simulink model "BANSHEE_20161130"  (Simulink 8.1)
settings: Solver=ode1  StartTime=0.0  StopTime=inf  FixedStep=Ts  MaxStep=1e-3  RelTol=1e-3
PostLoadFcn:
  | BANSHEE_init;
InitFcn:
  | BANSHEE_init;
values from neighbouring files (symbols this model uses):
  F1 = xlsread('F1_relay_banshee.xlsx')    [relay_settings_init.m]
  F2 = xlsread('F2_relay_banshee.xlsx')    [relay_settings_init.m]
  F3 = xlsread('F3_relay_banshee.xlsx')    [relay_settings_init.m]
  Ts = 100E-6    (= 0.0001)    [BANSHEE_init.m]
undefined symbols (not defined in the file or in its folder): cable_spec, fdesignblkfcn, Feeder1_lib, Feeder2_lib, Feeder3_lib, gcbh, generic_ethernet_cb, Left, relay_housing_lib, SM_UtilityService, SS_F1_RELAY_HOUSING, SS_F2_RELAY_HOUSING, SS_F3_RELAY_HOUSING, SS_Feeder1, SS_Feeder2, SS_Feeder3, type, utility_service_lib, V
libraries: breaker_lib x47, rtio_generic_modbus x43, relay_modbus_lib x42, cables_lib x38, transformer_lib x22, Load_lib x20, artemis x18, powerlib x18, rtio_opalrt_common x15, ssn_lib x15, rtlab x14, simulink x10
(part 3 of 5)

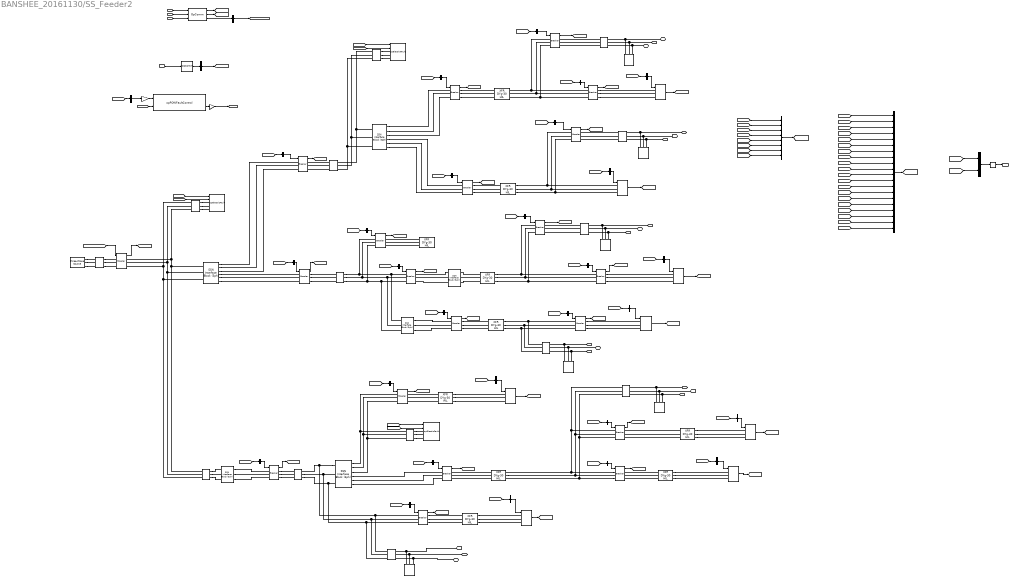
== system BANSHEE_20161130/SS_Feeder2 ==
  note: connect to F1
  note: connect to F1
  note: connect to F3
  note: connect to F3
  note: connect to F3
  note: BATT SYSTEM
  note: PV SYSTEM
  note: connect to F1
  note: % Copyright (c) 2016 Massachusetts Institute of Technology
      | % Permission is hereby granted, free of charge, to any person obtaining a copy of this
      | % software and associated documentation files (the "Software"), to deal in the Software
      | % without restriction, including without limitation the rights to use, copy, modify,
      | % merge, publish, distribute, sublicense, and/or sell copies of the Software, and to
      | % permit persons to whom the Software is furnished to do so, subject to the following
      | % conditions:
      | %
      | %
      | % The above copyright notice and this permission notice shall be included in
      | % all copies or substantial portions of the Software.
      | %
      | % THE SOFTWARE IS PROVIDED "AS IS", WITHOUT WARRANTY OF ANY KIND, EXPRESS OR IMPLIED,
      | % INCLUDING BUT NOT LIMITED TO THE WARRANTIES OF MERCHANTABILITY, FITNESS FOR A
      | % PARTICULAR PURPOSE AND NONINFRINGEMENT. IN NO EVENT SHALL THE AUTHORS OR COPYRIGHT
      | % HOLDERS BE LIABLE FOR ANY CLAIM, DAMAGES OR OTHER LIABILITY, WHETHER IN AN ACTION
      | % OF CONTRACT, TORT OR OTHERWISE, ARISING FROM, OUT OF OR IN CONNECTION WITH THE
      | % SOFTWARE OR THE USE OR OTHER DEALINGS IN THE SOFTWARE.
      | %
      | %
      | %%
  note: Point-on-wave synchronisation voltage (3-phase) in PU - Using 13.8 kV
  RELAY_IN : Inport
  LOAD_IN : Inport  Port=2
  SC_CMD : Inport  Port=3
  HWCtrl_CMD : Inport  Port=4
  1000 kVA1 : transformer_lib/XFR DYg-30 HIL  Rating=1000  Vp=13800  Vs=480  Z=5.56  XR=4.49
  1000 kVA2 : transformer_lib/XFR DYg-30 HIL  Rating=1000  Vp=13800  Vs=480  Z=5.56  XR=5.49
  1270 kvar inductor at 13.8kV  to cancel kvar produced by the stublines1 : powerlib/Elements/Three-Phase Parallel RLC Load  LConnTagsString=A|B|C  Configuration=Y (grounded)  NominalVoltage=13800  NominalFrequency=60  ActivePower=0  InductivePower=1270e3  CapacitivePower=0  Measurements=None  LoadType=constant Z
  1500 kVA : transformer_lib/XFR DYg-30 HIL  Rating=1500  Vp=13800  Vs=480  Z=5.56  XR=5.51
  2000 kVA2 : transformer_lib/XFR DYg-30 HIL  Rating=2000  Vp=13800  Vs=480  Z=5.75  XR=5.7
  2000 kVA3 : transformer_lib/XFR DYg-30 HIL  Rating=2000  Vp=13800  Vs=480  Z=5.75  XR=5.7
  2500 kVA : transformer_lib/XFR DYg-30 HIL  Rating=2500  Vp=13800  Vs=480  Z=5.56  XR=5.52
  2500 kVA1 : transformer_lib/XFR DYg-30 HIL  Rating=2500  Vp=13800  Vs=480  Z=5.56  XR=5.52
  346 kvar inductor at 4160V  to cancel kvar produced by the stublines5 : powerlib/Elements/Three-Phase Parallel RLC Load  LConnTagsString=A|B|C  Configuration=Y (grounded)  NominalVoltage=4160  NominalFrequency=60  ActivePower=0  InductivePower=346e3  CapacitivePower=0  Measurements=None  LoadType=constant Z
  3750 kVA : transformer_lib/XFR DYg-30 HIL  Rating=3750  Vp=13800  Vs=4160  Z=4.75  XR=11.4
  500 kVA : transformer_lib/XFR DYg-30 HIL  Rating=500  Vp=13800  Vs=208  Z=5  XR=4.9
  5000 kVA : transformer_lib/XFR DYg-30 HIL  Rating=5000  Vp=13800  Vs=480  Z=5.50  XR=5.44
  500kcmil_cable : cables_lib/500kcmil_cable  length=1  par_sets=1
  500kcmil_cable1 : cables_lib/500kcmil_cable  length=1  par_sets=1
  500kcmil_cable2 : cables_lib/500kcmil_cable  length=1  par_sets=1
  6 kvar inductor at 480V  to cancel kvar produced by the stublines1 : powerlib/Elements/Three-Phase Parallel RLC Load  LConnTagsString=A|B|C  Configuration=Y (grounded)  NominalVoltage=480  NominalFrequency=60  ActivePower=0  InductivePower=6e3  CapacitivePower=0  Measurements=None  LoadType=constant Z
  6 kvar inductor at 480V  to cancel kvar produced by the stublines2 : powerlib/Elements/Three-Phase Parallel RLC Load  LConnTagsString=A|B|C  Configuration=Y (grounded)  NominalVoltage=480  NominalFrequency=60  ActivePower=0  InductivePower=6e3  CapacitivePower=0  Measurements=None  LoadType=constant Z
  6 kvar inductor at 480V  to cancel kvar produced by the stublines3 : powerlib/Elements/Three-Phase Parallel RLC Load  LConnTagsString=A|B|C  Configuration=Y (grounded)  NominalVoltage=480  NominalFrequency=60  ActivePower=0  InductivePower=6e3  CapacitivePower=0  Measurements=None  LoadType=constant Z
  6 kvar inductor at 480V  to cancel kvar produced by the stublines4 : powerlib/Elements/Three-Phase Parallel RLC Load  LConnTagsString=A|B|C  Configuration=Y (grounded)  NominalVoltage=480  NominalFrequency=60  ActivePower=0  InductivePower=9e3  CapacitivePower=0  Measurements=None  LoadType=constant Z
  Bus Creator2 : BusCreator  Inputs=2
  Bus Creator3 : BusCreator  Inputs=8
  Bus Creator5 : BusCreator  Inputs=20
  Bus Selector : BusSelector  OutputSignals=Vabc_bus
  Bus Selector1 : BusSelector  OutputSignals=F2_CB_4
  Bus Selector10 : BusSelector  OutputSignals=I4
  Bus Selector11 : BusSelector  OutputSignals=F2_CB_11
  Bus Selector12 : BusSelector  OutputSignals=F2_CB_15
  Bus Selector13 : BusSelector  OutputSignals=F2_CB_3
  Bus Selector14 : BusSelector  OutputSignals=F2_CB_14
  Bus Selector15 : BusSelector  OutputSignals=F2_CB_17
  Bus Selector16 : BusSelector  OutputSignals=F2_CB_16
  Bus Selector17 : BusSelector  OutputSignals=F2_CB_13
  Bus Selector18 : BusSelector  OutputSignals=F2_CB_10
  Bus Selector19 : BusSelector  OutputSignals=F2_CB_9
  Bus Selector2 : BusSelector  OutputSignals=F2_CB_2
  Bus Selector20 : BusSelector  OutputSignals=F2_CB_12
  Bus Selector21 : BusSelector  OutputSignals=F2_CB_5
  Bus Selector22 : BusSelector  OutputSignals=F2_CB_7
  Bus Selector23 : BusSelector  OutputSignals=F2_CB_8
  Bus Selector24 : BusSelector  OutputSignals=F2_CB_6
  Bus Selector25 : BusSelector  OutputSignals=F2_CB_1
  Bus Selector26 : BusSelector  OutputSignals=F2_CB_18
  Bus Selector27 : BusSelector  OutputSignals=F2_CB_19
  Bus Selector28 : BusSelector  OutputSignals=fault_cmd
  Bus Selector29 : BusSelector  OutputSignals=SEL751_LogicTrip.F2.Logic_trip
  Bus Selector3 : BusSelector  OutputSignals=P5
  Bus Selector4 : BusSelector  OutputSignals=C4
  Bus Selector5 : BusSelector  OutputSignals=I5
  Bus Selector6 : BusSelector  OutputSignals=P2
  Bus Selector7 : BusSelector  OutputSignals=C3
  Bus Selector8 : BusSelector  OutputSignals=P3
  Bus Selector9 : BusSelector  OutputSignals=I3
  C1 : cables_lib/PI-Section  cable_spec=[cable_spec(11, :)]  line_length=10  parallel_sets=1
  C{2..4,204..206} (6 alike) : cables_lib/PI-Section  cable_spec=[cable_spec(6, :)]  line_length=10  parallel_sets=1
  C201 : cables_lib/PI-Section  cable_spec=[cable_spec(11, :)]  line_length=5500  parallel_sets=1
  C202 : cables_lib/PI-Section  cable_spec=[cable_spec(13, :)]  line_length=2000  parallel_sets=1
  C203 : cables_lib/PI-Section  cable_spec=[cable_spec(13, :)]  line_length=3000  parallel_sets=1
  Critical_3 : Load_lib/Dynamic_Load  V=460  Ts=Ts
  Critical_4 : Load_lib/Dynamic_Load  V=460  Ts=Ts
  F2_CB_{1..19} (19 alike) : breaker_lib/Breaker  Ts=Ts  mech_delay=cb_mech_delay
  F2_PCC : breaker_lib/Breaker  Ts=Ts  mech_delay=cb_mech_delay
  Interruptible_3 : Load_lib/Dynamic_Load  V=208  Ts=Ts
  Interruptible_4 : Load_lib/Dynamic_Load  V=460  Ts=Ts
  Interruptible_5 : Load_lib/Dynamic_Load  V=460  Ts=Ts
  Memory : Memory
  OpComm1 : rtlab/OpComm  nbport=3  groupe_acq=1  subsys_rate=0  st=0  Synchronization=on  Interpolation=on  Threshold=1.0  Missed_Data=off  Sim_Time=off  Samples=off  dynSigOut=off  from_console=0  warning_done=off  writeOpCommFile=off  Offset=off
  OpComm2 : rtlab/OpComm  nbport=1  groupe_acq=1  subsys_rate=0  st=0  Synchronization=on  Interpolation=on  Threshold=1.0  Missed_Data=off  Sim_Time=off  Samples=off  dynSigOut=off  from_console=1  warning_done=off  writeOpCommFile=off  Offset=off
  PI-Section1 : cables_lib/PI-Section  cable_spec=[cable_spec(13, :)]  line_length=500  parallel_sets=1
  Priority_2 : Load_lib/Dynamic_Load  V=460  Ts=Ts
  Priority_3 : Load_lib/Dynamic_Load  V=460  Ts=Ts
  Priority_5 : Load_lib/Dynamic_Load  V=460  Ts=Ts
  SSN Interface Block (3ph)1 : ssn_lib/SSN Interface Block (3ph)  nb_phase=3  nb_port=3  p1_type=V-type(Left)  p2_type=V-type (Right)  p3_type=V-type (Right)  p4_type=V-type(Left)  p5_type=V-type(Left)  p6_type=V-type(Left)  p7_type=V-type(Left)  p8_type=V-type(Left)  p9_type=V-type(Left)  p10_type=V-type(Left)  p11_type=V-type(Left)  p12_type=V-type(Left)  p13_type=V-type(Left)  p14_type=V-type(Left)  p15_type=V-type(Left)  p16_type=V-type(Left)  I_port_shunt_resistance=1e9
  SSN Interface Block (3ph)10 : ssn_lib/SSN Interface Block (3ph)  nb_phase=3  nb_port=2  p1_type=V-type(Left)  p2_type=V-type (Right)  p3_type=V-type(Left)  p4_type=V-type(Left)  p5_type=V-type(Left)  p6_type=V-type(Left)  p7_type=V-type(Left)  p8_type=V-type(Left)  p9_type=V-type(Left)  p10_type=V-type(Left)  p11_type=V-type(Left)  p12_type=V-type(Left)  p13_type=V-type(Left)  p14_type=V-type(Left)  p15_type=V-type(Left)  p16_type=V-type(Left)  I_port_shunt_resistance=1e9
  SSN Interface Block (3ph)2 : ssn_lib/SSN Interface Block (3ph)  nb_phase=3  nb_port=3  p1_type=V-type(Left)  p2_type=V-type (Right)  p3_type=V-type (Right)  p4_type=V-type(Left)  p5_type=V-type(Left)  p6_type=V-type(Left)  p7_type=V-type(Left)  p8_type=V-type(Left)  p9_type=V-type(Left)  p10_type=V-type(Left)  p11_type=V-type(Left)  p12_type=V-type(Left)  p13_type=V-type(Left)  p14_type=V-type(Left)  p15_type=V-type(Left)  p16_type=V-type(Left)  I_port_shunt_resistance=1e9
  SSN Interface Block (3ph)3 : ssn_lib/SSN Interface Block (3ph)  nb_phase=3  nb_port=2  p1_type=V-type(Left)  p2_type=V-type (Right)  p3_type=V-type(Left)  p4_type=V-type(Left)  p5_type=V-type(Left)  p6_type=V-type(Left)  p7_type=V-type(Left)  p8_type=V-type(Left)  p9_type=V-type(Left)  p10_type=V-type(Left)  p11_type=V-type(Left)  p12_type=V-type(Left)  p13_type=V-type(Left)  p14_type=V-type(Left)  p15_type=V-type(Left)  p16_type=V-type(Left)  I_port_shunt_resistance=1e9
  SSN Interface Block (3ph)4 : ssn_lib/SSN Interface Block (3ph)  nb_phase=3  nb_port=3  p1_type=V-type(Left)  p2_type=V-type (Right)  p3_type=V-type (Right)  p4_type=V-type(Left)  p5_type=V-type(Left)  p6_type=V-type(Left)  p7_type=V-type(Left)  p8_type=V-type(Left)  p9_type=V-type(Left)  p10_type=V-type(Left)  p11_type=V-type(Left)  p12_type=V-type(Left)  p13_type=V-type(Left)  p14_type=V-type(Left)  p15_type=V-type(Left)  p16_type=V-type(Left)  I_port_shunt_resistance=1e9
  SSN Interface Block (3ph)9 : ssn_lib/SSN Interface Block (3ph)  nb_phase=3  nb_port=2  p1_type=V-type(Left)  p2_type=V-type (Right)  p3_type=V-type(Left)  p4_type=V-type(Left)  p5_type=V-type(Left)  p6_type=V-type(Left)  p7_type=V-type(Left)  p8_type=V-type(Left)  p9_type=V-type(Left)  p10_type=V-type(Left)  p11_type=V-type(Left)  p12_type=V-type(Left)  p13_type=V-type(Left)  p14_type=V-type(Left)  p15_type=V-type(Left)  p16_type=V-type(Left)  I_port_shunt_resistance=1e9
  Three-Phase Source1 : powerlib/Electrical Sources/Three-Phase Source  Voltage=13800  PhaseAngle=0  Frequency=60  InternalConnection=Yg  SpecifyImpedance=on  Resistance=0.8929  Inductance=16.58e-3  ShortCircuitLevel=375e6  BaseVoltage=13800  XRratio=5.2  BusType=swing  Pref=0  Qref=0  Qmin=-inf  Qmax=inf
  a : Gain  Gain=1/(13800*sqrt(2/3))
  opElectricFault : artemis/Tools /POW faults/opElectricFault  FaultLocation=location 5  FaultResistance=0.0001  GroundResistance=0.0001  InitialStates=[0 0 0]  SnubberResistance=1e6  SnubberCapacitance=inf
  opElectricFault1 : artemis/Tools /POW faults/opElectricFault  FaultLocation=location 1  FaultResistance=0.0001  GroundResistance=0.0001  InitialStates=[0 0 0]  SnubberResistance=1e6  SnubberCapacitance=inf
  opElectricFault2 : artemis/Tools /POW faults/opElectricFault  FaultLocation=location 6  FaultResistance=0.0001  GroundResistance=0.0001  InitialStates=[0 0 0]  SnubberResistance=1e6  SnubberCapacitance=inf
  opPOWFaultControl1 : artemis/Tools /POW faults/opPOWFaultControl  Ts=Ts  usePLL=off  Fgrid=60  PLL_k=[180 3200 1]  vol_sel=1: rising zero-corssing  SyncPhase_menu=A  T_acq=0.8
  triggerFAULT : Gain
  A_CB_13 : PMIOPort  Port=1  Side=Right
  B_CB_13 : PMIOPort  Port=2  Side=Right
  C_CB_13 : PMIOPort  Port=3  Side=Right
  A_CB_17 : PMIOPort  Port=4  Side=Right
  B_CB_17 : PMIOPort  Port=5  Side=Right
  C_CB_17 : PMIOPort  Port=6  Side=Right
  A_CB_16 : PMIOPort  Port=7  Side=Right
  B_CB_16 : PMIOPort  Port=8  Side=Right
  C_CB_16 : PMIOPort  Port=9  Side=Right
  A_CB_9 : PMIOPort  Port=10  Side=Right
  B_CB_9 : PMIOPort  Port=11  Side=Right
  C_CB_9 : PMIOPort  Port=12  Side=Right
  A_CB_7 : PMIOPort  Port=13  Side=Right
  B_CB_7 : PMIOPort  Port=14  Side=Right
  C_CB_7 : PMIOPort  Port=15  Side=Right
  A_CB_1 : PMIOPort  Port=16  Side=Right
  B_CB_1 : PMIOPort  Port=17  Side=Right
  C_CB_1 : PMIOPort  Port=18  Side=Right
  DATA_OUT : Outport
  wires:
  LOAD_IN/1 -> OpComm1/1
  OpComm1/1 -> [LOAD_IN]
  [LOAD_IN] -> Bus Selector3/1
  [LOAD_IN] -> Bus Selector4/1
  [LOAD_IN] -> Bus Selector5/1
  [LOAD_IN] -> Bus Selector6/1
  [LOAD_IN] -> Bus Selector7/1
  [LOAD_IN] -> Bus Selector8/1
  [LOAD_IN] -> Bus Selector9/1
  [LOAD_IN] -> Bus Selector10/1
  Bus Selector3/1 -> Priority_5/1  "<P5>"
  Bus Selector4/1 -> Critical_4/1  "<C4>"
  Bus Selector5/1 -> Interruptible_5/1  "<I5>"
  Bus Selector6/1 -> Priority_2/1  "<P2>"
  Bus Selector7/1 -> Critical_3/1  "<C3>"
  Bus Selector8/1 -> Priority_3/1  "<P3>"
  Bus Selector10/1 -> Interruptible_4/1  "<I4>"
  Bus Selector9/1 -> Interruptible_3/1  "<I3>"
  Critical_4/1 -> [LOAD_C4]
  Priority_5/1 -> [LOAD_P5]
  Interruptible_5/1 -> [LOAD_I5]
  Priority_2/1 -> [LOAD_P2]
  Critical_3/1 -> [LOAD_C3]
  Interruptible_3/1 -> [LOAD_I3]
  Priority_3/1 -> [LOAD_P3]
  Interruptible_4/1 -> [LOAD_I4]
  [LOAD_C3] -> Bus Creator3/1  "F2_C3"
  Bus Creator3/1 -> [LOAD_DATA]  "LOAD"
  [LOAD_I4] -> Bus Creator3/4  "F2_I4"
  [LOAD_P2] -> Bus Creator3/6  "F2_P2"
  [LOAD_I5] -> Bus Creator3/5  "F2_I5"
  [LOAD_C4] -> Bus Creator3/2  "F2_C4"
  [LOAD_I3] -> Bus Creator3/3  "F2_I3"
  [LOAD_P3] -> Bus Creator3/7  "F2_P3"
  [LOAD_P5] -> Bus Creator3/8  "F2_P5"
  F2_CB_2/1 -> [F2_CB_2]
  F2_CB_1/1 -> [F2_CB_1]
  F2_CB_6/1 -> [F2_CB_6]
  F2_CB_7/1 -> [F2_CB_7]
  F2_CB_5/1 -> [F2_CB_5]
  F2_CB_8/1 -> [F2_CB_8]
  F2_CB_9/1 -> [F2_CB_9]
  F2_CB_3/1 -> [F2_CB_3]
  F2_CB_11/1 -> [F2_CB_11]
  F2_CB_15/1 -> [F2_CB_15]
  F2_CB_17/1 -> [F2_CB_17]
  F2_CB_14/1 -> [F2_CB_14]
  F2_CB_10/1 -> [F2_CB_10]
  F2_CB_13/1 -> [F2_CB_13]
  [F2_CB_1] -> Bus Creator5/1  "F2_CB_1"
  [F2_CB_2] -> Bus Creator5/2  "F2_CB_2"
  [F2_CB_3] -> Bus Creator5/3  "F2_CB_3"
  [F2_CB_6] -> Bus Creator5/6  "F2_CB_6"
  [F2_CB_4] -> Bus Creator5/4  "F2_CB_4"
  [F2_CB_9] -> Bus Creator5/9  "F2_CB_9"
  [F2_CB_7] -> Bus Creator5/7  "F2_CB_7"
  [F2_CB_11] -> Bus Creator5/11  "F2_CB_11"
  [F2_CB_14] -> Bus Creator5/14  "F2_CB_14"
  [F2_CB_5] -> Bus Creator5/5  "F2_CB_5"
  [F2_CB_8] -> Bus Creator5/8  "F2_CB_8"
  [F2_CB_12] -> Bus Creator5/12  "F2_CB_12"
  [F2_CB_10] -> Bus Creator5/10  "F2_CB_10"
  [F2_CB_13] -> Bus Creator5/13  "F2_CB_13"
  [F2_CB_15] -> Bus Creator5/15  "F2_CB_15"
  [F2_CB_16] -> Bus Creator5/16  "F2_CB_16"
  RELAY_IN/1 -> OpComm1/2
  OpComm1/2 -> [RELAY_IN]
  Bus Selector13/1 -> F2_CB_3/1  "<F2_CB_3>"
  [RELAY_IN] -> Bus Selector13/1
  [RELAY_IN] -> Bus Selector2/1
  [RELAY_IN] -> Bus Selector11/1
  [RELAY_IN] -> Bus Selector12/1
  [RELAY_IN] -> Bus Selector14/1
  [RELAY_IN] -> Bus Selector15/1
  [RELAY_IN] -> Bus Selector16/1
  [RELAY_IN] -> Bus Selector17/1
  [RELAY_IN] -> Bus Selector18/1
  [RELAY_IN] -> Bus Selector19/1
  [RELAY_IN] -> Bus Selector20/1
  [RELAY_IN] -> Bus Selector21/1
  [RELAY_IN] -> Bus Selector22/1
  [RELAY_IN] -> Bus Selector23/1
  [RELAY_IN] -> Bus Selector24/1
  [RELAY_IN] -> Bus Selector25/1
  Bus Selector2/1 -> F2_CB_2/1  "<F2_CB_2>"
  Bus Selector11/1 -> F2_CB_11/1  "<F2_CB_11>"
  Bus Selector18/1 -> F2_CB_10/1  "<F2_CB_10>"
  Bus Selector19/1 -> F2_CB_9/1  "<F2_CB_9>"
  Bus Selector17/1 -> F2_CB_13/1  "<F2_CB_13>"
  Bus Selector20/1 -> F2_CB_12/1  "<F2_CB_12>"
  Bus Selector14/1 -> F2_CB_14/1  "<F2_CB_14>"
  Bus Selector16/1 -> F2_CB_16/1  "<F2_CB_16>"
  Bus Selector12/1 -> F2_CB_15/1  "<F2_CB_15>"
  Bus Selector25/1 -> F2_CB_1/1  "<F2_CB_1>"
  Bus Selector21/1 -> F2_CB_5/1  "<F2_CB_5>"
  Bus Selector22/1 -> F2_CB_7/1  "<F2_CB_7>"
  Bus Selector24/1 -> F2_CB_6/1  "<F2_CB_6>"
  Bus Selector23/1 -> F2_CB_8/1  "<F2_CB_8>"
  [F2_CB_17] -> Bus Creator5/17  "F2_CB_17"
  Bus Selector15/1 -> F2_CB_17/1  "<F2_CB_17>"
  F2_CB_12/1 -> [F2_CB_12]
  F2_CB_16/1 -> [F2_CB_16]
  F2_PCC/1 -> [F2_PCC]
  [F2_PCC] -> Bus Creator5/20  "F2_PCC"
  F2_CB_4/1 -> [F2_CB_4]
  [RELAY_IN] -> Bus Selector1/1
  Bus Selector1/1 -> F2_CB_4/1  "<F2_CB_4>"
  F2_CB_18/1 -> [F2_CB_18]
  [RELAY_IN] -> Bus Selector26/1
  Bus Selector26/1 -> F2_CB_18/1  "<F2_CB_18>"
  [F2_CB_18] -> Bus Creator5/18  "F2_CB_18"
  [F2_CB_19] -> Bus Creator5/19  "F2_CB_19"
  F2_CB_19/1 -> [F2_CB_19]
  [RELAY_IN] -> Bus Selector27/1
  Bus Selector27/1 -> F2_CB_19/1  "<F2_CB_19>"
  [fault_cmd] -> opElectricFault/2
  [trigger] -> opElectricFault/1
  [fault_cmd] -> opElectricFault1/2
  [trigger] -> opElectricFault1/1
  [fault_cmd] -> opElectricFault2/2
  [trigger] -> opElectricFault2/1
  [fault_cmd] -> opPOWFaultControl1/2
  opPOWFaultControl1/2 -> triggerFAULT/1
  triggerFAULT/1 -> [trigger]  "triggerFAULTsig"
  [F2_PCC] -> Bus Selector/1
  Bus Selector/1 -> a/1  "<Vabc_bus>"
  a/1 -> opPOWFaultControl1/1
  SC_CMD/1 -> OpComm2/1
  Memory/1 -> DATA_OUT/1
  OpComm2/1 -> Bus Selector28/1
  Bus Selector28/1 -> [fault_cmd]  "<fault_cmd>"
  Bus Creator2/1 -> Memory/1
  Bus Creator5/1 -> [CB_DATA]
  [CB_DATA] -> Bus Creator2/1  "CB_DATA"
  [LOAD_DATA] -> Bus Creator2/2  "LOAD_DATA"
  [SEL751_F2_LogicTrip] -> F2_PCC/1
  HWCtrl_CMD/1 -> OpComm1/3
  Bus Selector29/1 -> [SEL751_F2_LogicTrip]  "<Logic_trip>"
  OpComm1/3 -> Bus Selector29/1
  connections:
  500kcmil_cable/LConn1 -- C203/RConn1 -- SSN Interface Block (3ph)2/LConn1
  500kcmil_cable/LConn2 -- SSN Interface Block (3ph)2/LConn2 -- C203/RConn2
  500kcmil_cable/LConn3 -- SSN Interface Block (3ph)2/LConn3 -- C203/RConn3
  F2_CB_13/LConn1 -- F2_CB_12/LConn1 -- 1000 kVA1/RConn1
  F2_CB_13/LConn2 -- 1000 kVA1/RConn2 -- F2_CB_12/LConn2
  F2_CB_13/LConn3 -- F2_CB_12/LConn3 -- 1000 kVA1/RConn3
  F2_CB_12/RConn3 -- Interruptible_5/LConn3
  F2_CB_12/RConn2 -- Interruptible_5/LConn2
  F2_CB_12/RConn1 -- Interruptible_5/LConn1
  1000 kVA1/LConn1 -- SSN Interface Block (3ph)9/RConn1
  1000 kVA1/LConn3 -- SSN Interface Block (3ph)9/RConn3
  1000 kVA1/LConn2 -- SSN Interface Block (3ph)9/RConn2
  3750 kVA/RConn2 -- F2_CB_4/LConn2 -- C3/LConn2 -- F2_CB_8/LConn2
  F2_CB_8/LConn3 -- C3/LConn3 -- F2_CB_4/LConn3 -- 3750 kVA/RConn3
  F2_CB_8/LConn1 -- C3/LConn1 -- F2_CB_4/LConn1 -- 3750 kVA/RConn1
  1000 kVA2/LConn3 -- F2_CB_8/RConn3
  1000 kVA2/LConn1 -- F2_CB_8/RConn1
  1000 kVA2/LConn2 -- F2_CB_8/RConn2
  500kcmil_cable2/LConn2 -- SSN Interface Block (3ph)1/RConn2 -- F2_CB_5/LConn2
  SSN Interface Block (3ph)4/RConn3 -- F2_CB_3/LConn3
  SSN Interface Block (3ph)4/RConn1 -- F2_CB_3/LConn1
  SSN Interface Block (3ph)4/RConn2 -- F2_CB_3/LConn2
  F2_CB_14/RConn3 -- 2000 kVA2/LConn3
  F2_CB_16/LConn2 -- 2000 kVA3/RConn2 -- F2_CB_18/LConn2
  F2_CB_14/RConn2 -- 2000 kVA2/LConn2
  F2_CB_6/RConn2 -- 500 kVA/LConn2
  SSN Interface Block (3ph)9/LConn3 -- F2_CB_10/RConn3
  F2_CB_9/RConn3 -- 2500 kVA1/LConn3
  SSN Interface Block (3ph)3/LConn3 -- F2_CB_10/LConn3 -- F2_CB_11/LConn3 -- C202/RConn3
  F2_CB_6/RConn3 -- 500 kVA/LConn3
  F2_CB_16/LConn3 -- 2000 kVA3/RConn3 -- F2_CB_18/LConn3
  5000 kVA/LConn2 -- F2_CB_11/RConn2
  Critical_4/LConn1 -- F2_CB_17/LConn1 -- 2000 kVA2/RConn1
  F2_CB_10/LConn2 -- SSN Interface Block (3ph)3/LConn2 -- F2_CB_11/LConn2 -- C202/RConn2
  SSN Interface Block (3ph)4/LConn1 -- 500kcmil_cable1/LConn3 -- F2_PCC/RConn1 -- C1/LConn1
  3750 kVA/LConn3 -- F2_CB_7/RConn3
  C203/LConn3 -- F2_CB_3/RConn3
  C203/LConn1 -- F2_CB_3/RConn1
  SSN Interface Block (3ph)9/LConn2 -- F2_CB_10/RConn2
  2500 kVA/LConn1 -- F2_CB_5/RConn1
  2500 kVA/LConn3 -- F2_CB_5/RConn3
  2500 kVA/LConn2 -- F2_CB_5/RConn2
  F2_CB_16/LConn1 -- F2_CB_18/LConn1 -- 2000 kVA3/RConn1
  SSN Interface Block (3ph)9/LConn1 -- F2_CB_10/RConn1
  F2_CB_14/RConn1 -- 2000 kVA2/LConn1
  F2_CB_15/RConn1 -- 2000 kVA3/LConn1
  Critical_4/LConn3 -- 2000 kVA2/RConn3 -- F2_CB_17/LConn3
  5000 kVA/LConn1 -- F2_CB_11/RConn1
  F2_CB_15/RConn3 -- 2000 kVA3/LConn3
  F2_CB_9/RConn1 -- 2500 kVA1/LConn1
  2500 kVA1/RConn2 -- C2/LConn2 -- F2_CB_19/LConn2
  C203/LConn2 -- F2_CB_3/RConn2
  5000 kVA/LConn3 -- F2_CB_11/RConn3
  Critical_4/LConn2 -- F2_CB_17/LConn2 -- 2000 kVA2/RConn2
  3750 kVA/LConn2 -- F2_CB_7/RConn2
  3750 kVA/LConn1 -- F2_CB_7/RConn1
  SSN Interface Block (3ph)3/LConn1 -- F2_CB_10/LConn1 -- F2_CB_11/LConn1 -- C202/RConn1
  F2_CB_15/RConn2 -- 2000 kVA3/LConn2
  F2_CB_6/RConn1 -- 500 kVA/LConn1
  SSN Interface Block (3ph)4/LConn2 -- 500kcmil_cable1/LConn2 -- F2_PCC/RConn2 -- C1/LConn2
  500kcmil_cable1/LConn1 -- C1/LConn3 -- SSN Interface Block (3ph)4/LConn3 -- F2_PCC/RConn3
  F2_CB_9/RConn2 -- 2500 kVA1/LConn2
  2500 kVA1/RConn1 -- C2/LConn1 -- F2_CB_19/LConn1
  2500 kVA1/RConn3 -- C2/LConn3 -- F2_CB_19/LConn3
  F2_CB_18/RConn1 -- Priority_5/LConn1
  F2_CB_18/RConn2 -- Priority_5/LConn2
  F2_CB_18/RConn3 -- Priority_5/LConn3
  F2_CB_19/RConn1 -- Priority_2/LConn1
  F2_CB_19/RConn2 -- Priority_2/LConn2
  F2_CB_19/RConn3 -- Priority_2/LConn3
  SSN Interface Block (3ph)3/RConn2 -- F2_CB_9/LConn2
  SSN Interface Block (3ph)3/RConn3 -- F2_CB_9/LConn3
  SSN Interface Block (3ph)3/RConn1 -- F2_CB_9/LConn1
  C204/LConn3 -- F2_CB_16/RConn3
  C204/LConn1 -- F2_CB_16/RConn1
  C204/LConn2 -- F2_CB_16/RConn2
  C_CB_16/RConn1 -- 6 kvar inductor at 480V  to cancel kvar produced by the stublines1/LConn3 -- C204/RConn3
  B_CB_16/RConn1 -- 6 kvar inductor at 480V  to cancel kvar produced by the stublines1/LConn2 -- C204/RConn2
  A_CB_16/RConn1 -- 6 kvar inductor at 480V  to cancel kvar produced by the stublines1/LConn1 -- C204/RConn1
  C205/LConn3 -- F2_CB_17/RConn3
  C205/LConn1 -- F2_CB_17/RConn1
  C205/LConn2 -- F2_CB_17/RConn2
  C_CB_17/RConn1 -- 6 kvar inductor at 480V  to cancel kvar produced by the stublines2/LConn3 -- C205/RConn3
  B_CB_17/RConn1 -- 6 kvar inductor at 480V  to cancel kvar produced by the stublines2/LConn2 -- C205/RConn2
  A_CB_17/RConn1 -- 6 kvar inductor at 480V  to cancel kvar produced by the stublines2/LConn1 -- C205/RConn1
  C206/LConn3 -- F2_CB_13/RConn3
  C206/LConn2 -- F2_CB_13/RConn2
  C206/LConn1 -- F2_CB_13/RConn1
  C_CB_13/RConn1 -- 6 kvar inductor at 480V  to cancel kvar produced by the stublines3/LConn3 -- C206/RConn3
  B_CB_13/RConn1 -- 6 kvar inductor at 480V  to cancel kvar produced by the stublines3/LConn2 -- C206/RConn2
  A_CB_13/RConn1 -- 6 kvar inductor at 480V  to cancel kvar produced by the stublines3/LConn1 -- C206/RConn1
  1500 kVA/RConn3 -- Priority_3/LConn3
  1500 kVA/RConn2 -- Priority_3/LConn2
  1500 kVA/RConn1 -- Priority_3/LConn1
  1500 kVA/LConn3 -- F2_CB_4/RConn3
  1500 kVA/LConn2 -- F2_CB_4/RConn2
  1500 kVA/LConn1 -- F2_CB_4/RConn1
  500kcmil_cable/RConn1 -- opElectricFault/LConn1
  500kcmil_cable/RConn2 -- opElectricFault/LConn2
  500kcmil_cable/RConn3 -- opElectricFault/LConn3
  500kcmil_cable1/RConn1 -- opElectricFault1/LConn1
  500kcmil_cable1/RConn2 -- opElectricFault1/LConn2
  500kcmil_cable1/RConn3 -- opElectricFault1/LConn3
  500kcmil_cable2/RConn1 -- opElectricFault2/LConn1
  500kcmil_cable2/RConn2 -- opElectricFault2/LConn2
  500kcmil_cable2/RConn3 -- opElectricFault2/LConn3
  SSN Interface Block (3ph)4/RConn5 -- F2_CB_2/LConn2
  SSN Interface Block (3ph)4/RConn6 -- F2_CB_2/LConn3
  SSN Interface Block (3ph)4/RConn4 -- F2_CB_2/LConn1
  F2_CB_2/RConn2 -- C202/LConn2
  F2_CB_2/RConn1 -- C202/LConn1
  F2_CB_2/RConn3 -- C202/LConn3
  SSN Interface Block (3ph)2/RConn1 -- F2_CB_15/LConn1
  SSN Interface Block (3ph)2/RConn2 -- F2_CB_15/LConn2
  SSN Interface Block (3ph)2/RConn3 -- F2_CB_15/LConn3
  SSN Interface Block (3ph)2/RConn6 -- F2_CB_14/LConn3
  SSN Interface Block (3ph)2/RConn5 -- F2_CB_14/LConn2
  SSN Interface Block (3ph)2/RConn4 -- F2_CB_14/LConn1
  500kcmil_cable2/LConn3 -- F2_CB_5/LConn3 -- SSN Interface Block (3ph)1/RConn3
  500kcmil_cable2/LConn1 -- F2_CB_5/LConn1 -- SSN Interface Block (3ph)1/RConn1
  F2_CB_1/RConn1 -- C201/LConn1
  F2_CB_1/RConn2 -- C201/LConn2
  F2_CB_1/RConn3 -- C201/LConn3
  C201/RConn2 -- C4/LConn2 -- F2_CB_6/LConn2 -- SSN Interface Block (3ph)1/LConn2
  SSN Interface Block (3ph)1/LConn1 -- C4/LConn1 -- F2_CB_6/LConn1 -- C201/RConn1
  C201/RConn3 -- C4/LConn3 -- F2_CB_6/LConn3 -- SSN Interface Block (3ph)1/LConn3
  SSN Interface Block (3ph)1/RConn4 -- F2_CB_7/LConn1
  SSN Interface Block (3ph)1/RConn5 -- F2_CB_7/LConn2
  SSN Interface Block (3ph)1/RConn6 -- F2_CB_7/LConn3
  SSN Interface Block (3ph)10/RConn1 -- F2_CB_1/LConn1
  SSN Interface Block (3ph)10/RConn2 -- F2_CB_1/LConn2
  SSN Interface Block (3ph)10/RConn3 -- F2_CB_1/LConn3
  C1/RConn2 -- SSN Interface Block (3ph)10/LConn2
  C1/RConn1 -- SSN Interface Block (3ph)10/LConn1
  C1/RConn3 -- SSN Interface Block (3ph)10/LConn3
  2500 kVA/RConn1 -- Critical_3/LConn1
  2500 kVA/RConn3 -- Critical_3/LConn3
  2500 kVA/RConn2 -- Critical_3/LConn2
  1000 kVA2/RConn1 -- Interruptible_4/LConn1
  1000 kVA2/RConn2 -- Interruptible_4/LConn2
  1000 kVA2/RConn3 -- Interruptible_4/LConn3
  500 kVA/RConn2 -- Interruptible_3/LConn2
  500 kVA/RConn3 -- Interruptible_3/LConn3
  500 kVA/RConn1 -- Interruptible_3/LConn1
  A_CB_9/RConn1 -- 6 kvar inductor at 480V  to cancel kvar produced by the stublines4/LConn1 -- C2/RConn1
  C_CB_9/RConn1 -- 6 kvar inductor at 480V  to cancel kvar produced by the stublines4/LConn3 -- C2/RConn3
  B_CB_9/RConn1 -- 6 kvar inductor at 480V  to cancel kvar produced by the stublines4/LConn2 -- C2/RConn2
  C_CB_7/RConn1 -- 346 kvar inductor at 4160V  to cancel kvar produced by the stublines5/LConn3 -- C3/RConn3
  A_CB_7/RConn1 -- C3/RConn1 -- 346 kvar inductor at 4160V  to cancel kvar produced by the stublines5/LConn1
  B_CB_7/RConn1 -- 346 kvar inductor at 4160V  to cancel kvar produced by the stublines5/LConn2 -- C3/RConn2
  A_CB_1/RConn1 -- 1270 kvar inductor at 13.8kV  to cancel kvar produced by the stublines1/LConn1 -- C4/RConn1
  C_CB_1/RConn1 -- 1270 kvar inductor at 13.8kV  to cancel kvar produced by the stublines1/LConn3 -- C4/RConn3
  B_CB_1/RConn1 -- 1270 kvar inductor at 13.8kV  to cancel kvar produced by the stublines1/LConn2 -- C4/RConn2
  Three-Phase Source1/RConn2 -- PI-Section1/LConn2
  Three-Phase Source1/RConn3 -- PI-Section1/LConn3
  Three-Phase Source1/RConn1 -- PI-Section1/LConn1
  PI-Section1/RConn2 -- F2_PCC/LConn2
  PI-Section1/RConn3 -- F2_PCC/LConn3
  PI-Section1/RConn1 -- F2_PCC/LConn1

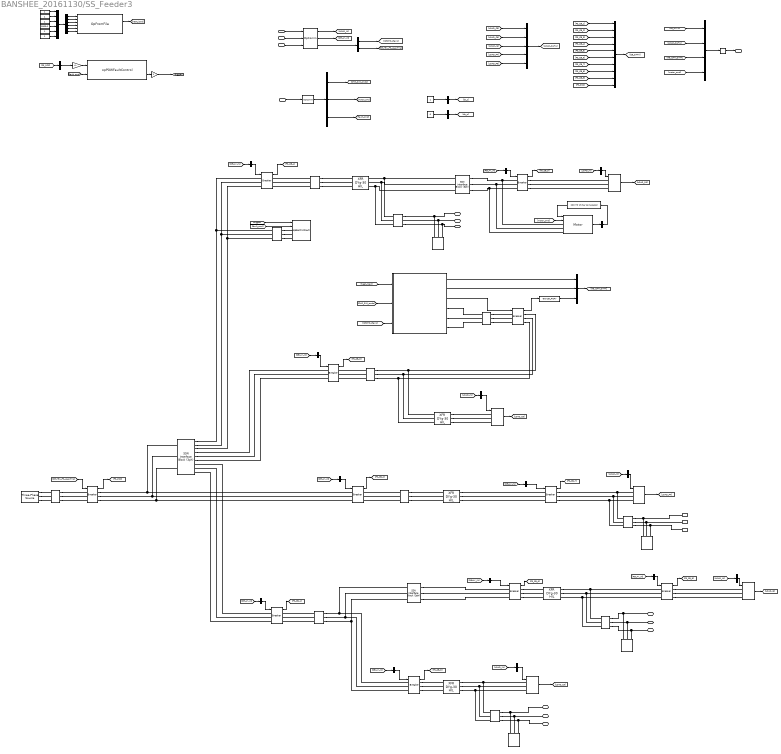
== system BANSHEE_20161130/SS_Feeder3 ==
  note: Signal for this Cb will come from a SEL relay
  note: connect to F2
  note: connect to F2
  note: connect to F2
  note: connect to F1
  note: % Copyright (c) 2016 Massachusetts Institute of Technology
      | % Permission is hereby granted, free of charge, to any person obtaining a copy of this
      | % software and associated documentation files (the "Software"), to deal in the Software
      | % without restriction, including without limitation the rights to use, copy, modify,
      | % merge, publish, distribute, sublicense, and/or sell copies of the Software, and to
      | % permit persons to whom the Software is furnished to do so, subject to the following
      | % conditions:
      | %
      | %
      | % The above copyright notice and this permission notice shall be included in
      | % all copies or substantial portions of the Software.
      | %
      | % THE SOFTWARE IS PROVIDED "AS IS", WITHOUT WARRANTY OF ANY KIND, EXPRESS OR IMPLIED,
      | % INCLUDING BUT NOT LIMITED TO THE WARRANTIES OF MERCHANTABILITY, FITNESS FOR A
      | % PARTICULAR PURPOSE AND NONINFRINGEMENT. IN NO EVENT SHALL THE AUTHORS OR COPYRIGHT
      | % HOLDERS BE LIABLE FOR ANY CLAIM, DAMAGES OR OTHER LIABILITY, WHETHER IN AN ACTION
      | % OF CONTRACT, TORT OR OTHERWISE, ARISING FROM, OUT OF OR IN CONNECTION WITH THE
      | % SOFTWARE OR THE USE OR OTHER DEALINGS IN THE SOFTWARE.
      | %
      | %
      | %%
  note: Point-on-wave synchronisation voltage (3-phase) in PU - Using 13.8 kV
  RELAY_IN : Inport
  LOAD_IN : Inport  Port=2
  SC_CMD : Inport  Port=3
  HWCtrl_CMD : Inport  Port=4
  1000 kVA : transformer_lib/XFR DYg-30 HIL  Rating=1000  Vp=13800  Vs=480  Z=5.56  XR=5.49
  1000 kVA1 : transformer_lib/XFR DYg-30 HIL  Rating=1000  Vp=13800  Vs=480  Z=5.56  XR=5.49
  200 HP chiller compressor : Load_lib/200 HP chiller compressor
  2000 kVA : transformer_lib/XFR DYg-30 HIL  Rating=2000  Vp=13800  Vs=480  Z=5.75  XR=5.7
  2000 kVA1 : transformer_lib/XFR DYg-30 HIL  Rating=2000  Vp=13800  Vs=480  Z=5.75  XR=5.7
  2500 kVA : transformer_lib/XFR DYg-30 HIL  Rating=2500  Vp=13800  Vs=480  Z=5.75  XR=6.6
  5 kvar inductor at 480V  to cancel kvar produced by the stublines : powerlib/Elements/Three-Phase Parallel RLC Load  LConnTagsString=A|B|C  Configuration=Y (grounded)  NominalVoltage=480  NominalFrequency=60  ActivePower=0  InductivePower=5e3  CapacitivePower=0  Measurements=None  LoadType=constant Z
  500kcmil_cable : cables_lib/500kcmil_cable  length=1  par_sets=1
  6 kvar inductor at 480V  to cancel kvar produced by the stublines1 : powerlib/Elements/Three-Phase Parallel RLC Load  LConnTagsString=A|B|C  Configuration=Y (grounded)  NominalVoltage=480  NominalFrequency=60  ActivePower=0  InductivePower=6e3  CapacitivePower=0  Measurements=None  LoadType=constant Z
  6 kvar inductor at 480V  to cancel kvar produced by the stublines2 : powerlib/Elements/Three-Phase Parallel RLC Load  LConnTagsString=A|B|C  Configuration=Y (grounded)  NominalVoltage=480  NominalFrequency=60  ActivePower=0  InductivePower=6e3  CapacitivePower=0  Measurements=None  LoadType=constant Z
  6 kvar inductor at 480V  to cancel kvar produced by the stublines3 : powerlib/Elements/Three-Phase Parallel RLC Load  LConnTagsString=A|B|C  Configuration=Y (grounded)  NominalVoltage=480  NominalFrequency=60  ActivePower=0  InductivePower=6e3  CapacitivePower=0  Measurements=None  LoadType=constant Z
  Bus Creator : BusCreator  Inputs=1
  Bus Creator1 : BusCreator  Inputs=1
  Bus Creator2 : BusCreator
  Bus Creator3 : BusCreator  Inputs=5
  Bus Creator5 : BusCreator  Inputs=10
  Bus Creator6 : BusCreator  Inputs=3
  Bus Selector : BusSelector  OutputSignals=Vabc_bus
  Bus Selector1 : BusSelector  OutputSignals=F3_CB_4
  Bus Selector10 : BusSelector  OutputSignals=F3_CB_5
  Bus Selector11 : BusSelector  OutputSignals=P6
  Bus Selector12 : BusSelector  OutputSignals=F3_CB_9
  Bus Selector13 : BusSelector  OutputSignals=F3_CB_3
  Bus Selector14 : BusSelector  OutputSignals=F3_CB_8
  Bus Selector15 : BusSelector  OutputSignals=IO ctrl.16 DOUT GR3.CHP_SIM_Cmds,motor_ONOFF.F3_motor_ONOFF,fault_cmd
  Bus Selector16 : BusSelector  OutputSignals=NGCHP_Gen1,SEL751_LogicTrip.F3.Logic_trip
  Bus Selector17 : BusSelector  OutputSignals=RPM
  Bus Selector2 : BusSelector  OutputSignals=C6
  Bus Selector3 : BusSelector  OutputSignals=P4
  Bus Selector4 : BusSelector  OutputSignals=I6
  Bus Selector5 : BusSelector  OutputSignals=C5
  Bus Selector6 : BusSelector  OutputSignals=F3_CB_2
  Bus Selector7 : BusSelector  OutputSignals=F3_CB_7
  Bus Selector8 : BusSelector  OutputSignals=F3_CB_6
  Bus Selector9 : BusSelector  OutputSignals=F3_CB_1
  C{1..4} (4 alike) : cables_lib/PI-Section  cable_spec=[cable_spec(13, :)]  line_length=10  parallel_sets=1
  C301 : cables_lib/PI-Section  cable_spec=[cable_spec(13, :)]  line_length=2500  parallel_sets=1
  C302 : cables_lib/PI-Section  cable_spec=[cable_spec(11, :)]  line_length=2000  parallel_sets=1
  C303 : cables_lib/PI-Section  cable_spec=[cable_spec(13, :)]  line_length=2000  parallel_sets=1
  C304 : cables_lib/PI-Section  cable_spec=[cable_spec(11, :)]  line_length=1500  parallel_sets=2
  CB closed : Constant
  CB open : Constant  Value=0
  Critical_5 : Load_lib/Dynamic_Load  V=460  Ts=Ts
  Critical_6 : Load_lib/Dynamic_Load  V=460  Ts=Ts
  Demux2 : Demux  Outputs=6
  F3_CB_{1..9} (9 alike) : breaker_lib/Breaker  Ts=Ts  mech_delay=cb_mech_delay
  F3_GCB : breaker_lib/Breaker  Ts=Ts  mech_delay=cb_mech_delay
  F3_PCC : breaker_lib/Breaker  Ts=Ts  mech_delay=cb_mech_delay
  Genset_PQFV : PQFV_lib/Genset_PQFV  VRMSLL=13800
  HWController_3.5MVA_NGCHP : Subsystem  AncestorBlock=HWController_NGCHP_Genset_3p5MVA_lib/HWController_3.5MVA_NGCHP
  "Interpolation " : Constant
  Interruptible_6 : Load_lib/Dynamic_Load  V=460  Ts=Ts
  Memory : Memory
  Motor : Motor_InductionMachine_lib/Motor
  Mux : Mux  Inputs=6
  OpComm1 : rtlab/OpComm  nbport=3  groupe_acq=1  subsys_rate=0  st=0  Synchronization=on  Interpolation=on  Threshold=1.0  Missed_Data=off  Sim_Time=off  Samples=off  dynSigOut=off  from_console=0  warning_done=off  writeOpCommFile=off  Offset=off
  OpComm2 : rtlab/OpComm  nbport=1  groupe_acq=1  subsys_rate=0  st=0  Synchronization=on  Interpolation=on  Threshold=1.0  Missed_Data=off  Sim_Time=off  Samples=off  dynSigOut=off  from_console=1  warning_done=off  writeOpCommFile=off  Offset=off
  OpFromFile : rtlab/DataLogging/OpFromFile  filename_mode=Static (same filename all the time)  reload_mode=Next time model is paused (Real-Time)  init_file_id=0  filename=HeatLoad.mat  rtpath='./'  nrtpath='.\'  sample_time=Ts
  PI-Section1 : cables_lib/PI-Section  cable_spec=[cable_spec(13, :)]  line_length=500  parallel_sets=1
  PI-Section2 : cables_lib/PI-Section  cable_spec=[cable_spec(11, :)]  line_length=2000  parallel_sets=1
  Priority_4 : Load_lib/Dynamic_Load  V=460  Ts=Ts
  Priority_6 : Load_lib/Dynamic_Load  V=460  Ts=Ts
  "Repetative " : Constant
  SSN Interface Block (3ph)1 : ssn_lib/SSN Interface Block (3ph)  nb_phase=3  nb_port=2  p1_type=V-type(Left)  p2_type=V-type (Right)  p3_type=V-type(Left)  p4_type=V-type(Left)  p5_type=V-type(Left)  p6_type=V-type(Left)  p7_type=V-type(Left)  p8_type=V-type(Left)  p9_type=V-type(Left)  p10_type=V-type(Left)  p11_type=V-type(Left)  p12_type=V-type(Left)  p13_type=V-type(Left)  p14_type=V-type(Left)  p15_type=V-type(Left)  p16_type=V-type(Left)  I_port_shunt_resistance=1e9
  SSN Interface Block (3ph)2 : ssn_lib/SSN Interface Block (3ph)  nb_phase=3  nb_port=2  p1_type=V-type(Left)  p2_type=V-type (Right)  p3_type=V-type(Left)  p4_type=V-type(Left)  p5_type=V-type(Left)  p6_type=V-type(Left)  p7_type=V-type(Left)  p8_type=V-type(Left)  p9_type=V-type(Left)  p10_type=V-type(Left)  p11_type=V-type(Left)  p12_type=V-type(Left)  p13_type=V-type(Left)  p14_type=V-type(Left)  p15_type=V-type(Left)  p16_type=V-type(Left)  I_port_shunt_resistance=1e9
  SSN Interface Block (3ph)5 : ssn_lib/SSN Interface Block (3ph)  nb_phase=3  nb_port=4  p1_type=V-type(Left)  p2_type=V-type (Right)  p3_type=V-type (Right)  p4_type=V-type (Right)  p5_type=V-type(Left)  p6_type=V-type(Left)  p7_type=V-type(Left)  p8_type=V-type(Left)  p9_type=V-type(Left)  p10_type=V-type(Left)  p11_type=V-type(Left)  p12_type=V-type(Left)  p13_type=V-type(Left)  p14_type=V-type(Left)  p15_type=V-type(Left)  p16_type=V-type(Left)  I_port_shunt_resistance=1e9
  "Start_Index " : Constant
  "State " : Constant
  "Stop_Index " : Constant  Value=1800-1
  Three-Phase Source1 : powerlib/Electrical Sources/Three-Phase Source  Voltage=13800  PhaseAngle=0  Frequency=60  InternalConnection=Yg  SpecifyImpedance=on  Resistance=0.8929  Inductance=16.58e-3  ShortCircuitLevel=350e6  BaseVoltage=13800  XRratio=4.7  BusType=swing  Pref=0  Qref=0  Qmin=-inf  Qmax=inf
  "Time_Scale_Factor " : Constant
  a : Gain  Gain=1/(13800*sqrt(2/3))
  opElectricFault : artemis/Tools /POW faults/opElectricFault  FaultLocation=location 4  FaultResistance=0.0001  GroundResistance=0.0001  InitialStates=[0 0 0]  SnubberResistance=1e6  SnubberCapacitance=inf
  opPOWFaultControl1 : artemis/Tools /POW faults/opPOWFaultControl  Ts=Ts  usePLL=off  Fgrid=60  PLL_k=[180 3200 1]  vol_sel=1: rising zero-corssing  SyncPhase_menu=A  T_acq=0.8
  triggerFAULT : Gain
  A_CB_4 : PMIOPort  Port=1  Side=Right
  B_CB_4 : PMIOPort  Port=2  Side=Right
  C_CB_4 : PMIOPort  Port=3  Side=Right
  A_CB_5 : PMIOPort  Port=4  Side=Right
  B_CB_5 : PMIOPort  Port=5  Side=Right
  C_CB_5 : PMIOPort  Port=6  Side=Right
  A_CB_6 : PMIOPort  Port=7  Side=Right
  B_CB_6 : PMIOPort  Port=8  Side=Right
  C_CB_6 : PMIOPort  Port=9  Side=Right
  A_CB_7 : PMIOPort  Port=10  Side=Right
  B_CB_7 : PMIOPort  Port=11  Side=Right
  C_CB_7 : PMIOPort  Port=12  Side=Right
  DATA_OUT : Outport
  wires:
  CB closed/1 -> Bus Creator/1  "Logic_trip"
  Bus Creator/1 -> [cb_c]
  Bus Creator1/1 -> [cb_o]
  Bus Selector1/1 -> F3_CB_4/1  "<F3_CB_4>"
  CB open/1 -> Bus Creator1/1  "Logic_trip"
  LOAD_IN/1 -> OpComm1/1
  OpComm1/1 -> [LOAD_IN]
  [LOAD_IN] -> Bus Selector2/1
  [LOAD_IN] -> Bus Selector3/1
  [LOAD_IN] -> Bus Selector4/1
  [LOAD_IN] -> Bus Selector5/1
  Bus Selector2/1 -> Critical_6/1  "<C6>"
  Bus Selector3/1 -> Priority_4/1  "<P4>"
  Bus Selector4/1 -> Interruptible_6/1  "<I6>"
  Bus Selector5/1 -> Critical_5/1  "<C5>"
  Critical_6/1 -> [LOAD_C6]
  Priority_4/1 -> [LOAD_P4]
  Interruptible_6/1 -> [LOAD_I6]
  Critical_5/1 -> [LOAD_C5]
  [LOAD_C6] -> Bus Creator3/2  "F3_C6"
  [LOAD_C5] -> Bus Creator3/1  "F3_C5"
  [LOAD_I6] -> Bus Creator3/3  "F3_I6"
  [LOAD_P4] -> Bus Creator3/4  "F3_P4"
  Bus Creator3/1 -> [LOAD_DATA]  "LOAD"
  F3_CB_4/1 -> [F3_CB_4]
  F3_CB_3/1 -> [F3_CB_3]
  F3_CB_2/1 -> [F3_CB_2]
  F3_CB_6/1 -> [F3_CB_6]
  F3_CB_1/1 -> [F3_CB_1]
  F3_CB_5/1 -> [F3_CB_5]
  [F3_CB_1] -> Bus Creator5/1  "F3_CB_1"
  [F3_CB_5] -> Bus Creator5/5  "F3_CB_5"
  [F3_CB_7] -> Bus Creator5/7  "F3_CB_7"
  [F3_CB_6] -> Bus Creator5/6  "F3_CB_6"
  [F3_CB_3] -> Bus Creator5/3  "F3_CB_3"
  [F3_CB_2] -> Bus Creator5/2  "F3_CB_2"
  [F3_CB_4] -> Bus Creator5/4  "F3_CB_4"
  Bus Creator5/1 -> [CB_DATA]
  [RELAY_IN] -> Bus Selector1/1
  RELAY_IN/1 -> OpComm1/2
  OpComm1/2 -> [RELAY_IN]
  Bus Selector6/1 -> F3_CB_2/1  "<F3_CB_2>"
  [RELAY_IN] -> Bus Selector6/1
  Bus Selector7/1 -> F3_CB_7/1  "<F3_CB_7>"
  [RELAY_IN] -> Bus Selector7/1
  Bus Selector8/1 -> F3_CB_6/1  "<F3_CB_6>"
  [RELAY_IN] -> Bus Selector8/1
  Bus Selector9/1 -> F3_CB_1/1  "<F3_CB_1>"
  [RELAY_IN] -> Bus Selector9/1
  Bus Selector10/1 -> F3_CB_5/1  "<F3_CB_5>"
  [RELAY_IN] -> Bus Selector10/1
  Bus Selector13/1 -> F3_CB_3/1  "<F3_CB_3>"
  [RELAY_IN] -> Bus Selector13/1
  [SEL751_F3_LogicTrip] -> F3_PCC/1
  F3_CB_7/1 -> [F3_CB_7]
  F3_PCC/1 -> [F3_PCC]
  [F3_PCC] -> Bus Creator5/10  "F3_PCC"
  [LOAD_IN] -> Bus Selector11/1
  Bus Selector11/1 -> Priority_6/1  "<P6>"
  Priority_6/1 -> [LOAD_P6]
  [LOAD_P6] -> Bus Creator3/5  "F3_P6"
  F3_CB_9/1 -> [F3_CB_9]
  Bus Selector12/1 -> F3_CB_9/1  "<F3_CB_9>"
  [RELAY_IN] -> Bus Selector12/1
  F3_CB_8/1 -> [F3_CB_8]
  Bus Selector14/1 -> F3_CB_8/1  "<F3_CB_8>"
  [RELAY_IN] -> Bus Selector14/1
  [F3_CB_8] -> Bus Creator5/8  "F3_CB_8"
  [F3_CB_9] -> Bus Creator5/9  "F3_CB_9"
  [fault_cmd] -> opPOWFaultControl1/2
  opPOWFaultControl1/2 -> triggerFAULT/1
  triggerFAULT/1 -> [trigger]  "triggerFAULTsig"
  [F3_PCC] -> Bus Selector/1
  Bus Selector/1 -> a/1  "<Vabc_bus>"
  a/1 -> opPOWFaultControl1/1
  [fault_cmd] -> opElectricFault/2
  [trigger] -> opElectricFault/1
  SC_CMD/1 -> OpComm2/1
  Memory/1 -> DATA_OUT/1
  "Start_Index "/1 -> Mux/3
  "Time_Scale_Factor "/1 -> Mux/5
  "State "/1 -> Mux/1
  Demux2/1 -> OpFromFile/1
  Demux2/4 -> OpFromFile/4
  OpFromFile/2 -> [heat_load]  "Heat Load MBtu/hr"
  Demux2/5 -> OpFromFile/5
  "Repetative "/1 -> Mux/2
  Demux2/3 -> OpFromFile/3
  Demux2/6 -> OpFromFile/6
  Demux2/2 -> OpFromFile/2
  Mux/1 -> Demux2/1
  "Interpolation "/1 -> Mux/6
  "Stop_Index "/1 -> Mux/4
  Bus Selector15/2 -> [motor_cmd]  "<F3_motor_ONOFF>"
  OpComm2/1 -> Bus Selector15/1
  Bus Selector15/3 -> [fault_cmd]  "<fault_cmd>"
  F3_GCB/1 -> Genset_PQFV/1
  Genset_PQFV/1 -> Bus Creator6/3  "NG_CHP_GCB"
  HWController_3.5MVA_NGCHP/2(Generator Data) -> Bus Creator6/2  "Gen1_meas"
  HWController_3.5MVA_NGCHP/1(Out1) -> Bus Creator6/1  "CHPData"
  [CHP_SIM_cmds] -> HWController_3.5MVA_NGCHP/2(In2)
  Bus Creator6/1 -> [NG_CHP_DATA]
  [NGCHP_Gen1] -> HWController_3.5MVA_NGCHP/3(HWControllerBias)
  HWController_3.5MVA_NGCHP/3(GCB Control) -> F3_GCB/1
  [heat_load] -> HWController_3.5MVA_NGCHP/1(In1)
  HWCtrl_CMD/1 -> OpComm1/3
  OpComm1/3 -> Bus Selector16/1
  Bus Selector16/1 -> [NGCHP_Gen1]  "<NGCHP_Gen1>"
  Bus Creator2/1 -> Memory/1
  [CB_DATA] -> Bus Creator2/1  "CB_DATA"
  [LOAD_DATA] -> Bus Creator2/2  "LOAD_DATA"
  [NG_CHP_DATA] -> Bus Creator2/3  "NG_CHP_DATA"
  Bus Selector15/1 -> [CHP_SIM_cmds]  "<CHP_SIM_Cmds>"
  [motor_cmd] -> Motor/2
  Motor/1 -> Bus Selector17/1
  Bus Selector17/1 -> 200 HP chiller compressor/1  "<RPM>"
  200 HP chiller compressor/1 -> Motor/1
  [motor_cmd] -> Bus Creator2/4  "MOTOR_ONOFF"
  Bus Selector16/2 -> [SEL751_F3_LogicTrip]  "<Logic_trip>"
  connections:
  F3_CB_5/LConn1 -- C301/RConn1 -- SSN Interface Block (3ph)1/LConn1
  F3_CB_6/RConn3 -- 2000 kVA1/LConn3
  C301/LConn2 -- F3_CB_1/RConn2
  F3_CB_5/LConn3 -- C301/RConn3 -- SSN Interface Block (3ph)1/LConn3
  C301/LConn3 -- F3_CB_1/RConn3
  C304/LConn1 -- F3_CB_2/RConn1
  C302/RConn3 -- F3_GCB/RConn3 -- 1000 kVA1/LConn3
  C302/LConn2 -- F3_CB_3/RConn2
  C302/RConn1 -- F3_GCB/RConn1 -- 1000 kVA1/LConn1
  F3_CB_6/RConn2 -- 2000 kVA1/LConn2
  C302/RConn2 -- F3_GCB/RConn2 -- 1000 kVA1/LConn2
  C301/LConn1 -- F3_CB_1/RConn1
  F3_CB_5/RConn2 -- 2000 kVA/LConn2
  C302/LConn3 -- F3_CB_3/RConn3
  F3_CB_5/LConn2 -- C301/RConn2 -- SSN Interface Block (3ph)1/LConn2
  C304/LConn2 -- F3_CB_2/RConn2
  F3_CB_6/RConn1 -- 2000 kVA1/LConn1
  C302/LConn1 -- F3_CB_3/RConn1
  F3_CB_5/RConn1 -- 2000 kVA/LConn1
  F3_CB_5/RConn3 -- 2000 kVA/LConn3
  C304/LConn3 -- F3_CB_2/RConn3
  F3_CB_7/RConn1 -- C3/LConn1 -- Priority_4/LConn1
  F3_CB_7/RConn3 -- C3/LConn3 -- Priority_4/LConn3
  F3_CB_7/RConn2 -- C3/LConn2 -- Priority_4/LConn2
  2000 kVA1/RConn1 -- C2/LConn1 -- F3_CB_8/LConn1
  F3_CB_8/LConn3 -- C2/LConn3 -- 2000 kVA1/RConn3
  2000 kVA1/RConn2 -- C2/LConn2 -- F3_CB_8/LConn2
  2000 kVA/RConn1 -- C1/LConn1 -- Critical_5/LConn1
  2000 kVA/RConn3 -- C1/LConn3 -- Critical_5/LConn3
  2000 kVA/RConn2 -- C1/LConn2 -- Critical_5/LConn2
  SSN Interface Block (3ph)2/LConn1 -- C4/LConn1 -- 2500 kVA/RConn1
  SSN Interface Block (3ph)2/LConn3 -- C4/LConn3 -- 2500 kVA/RConn3
  SSN Interface Block (3ph)2/LConn2 -- C4/LConn2 -- 2500 kVA/RConn2
  C304/RConn2 -- 1000 kVA/LConn2
  C304/RConn3 -- 1000 kVA/LConn3
  C304/RConn1 -- 1000 kVA/LConn1
  1000 kVA/RConn3 -- F3_CB_7/LConn3
  1000 kVA/RConn2 -- F3_CB_7/LConn2
  1000 kVA/RConn1 -- F3_CB_7/LConn1
  F3_CB_9/RConn1 -- Priority_6/LConn1
  F3_CB_9/RConn2 -- Priority_6/LConn2
  F3_CB_9/RConn3 -- Priority_6/LConn3
  F3_CB_8/RConn1 -- Interruptible_6/LConn1
  F3_CB_8/RConn2 -- Interruptible_6/LConn2
  F3_CB_8/RConn3 -- Interruptible_6/LConn3
  SSN Interface Block (3ph)5/RConn1 -- 500kcmil_cable/LConn1 -- F3_CB_4/LConn1
  SSN Interface Block (3ph)5/RConn3 -- 500kcmil_cable/LConn3 -- F3_CB_4/LConn3
  SSN Interface Block (3ph)5/RConn2 -- 500kcmil_cable/LConn2 -- F3_CB_4/LConn2
  SSN Interface Block (3ph)5/RConn4 -- F3_CB_3/LConn1
  SSN Interface Block (3ph)5/RConn6 -- F3_CB_3/LConn3
  SSN Interface Block (3ph)5/RConn5 -- F3_CB_3/LConn2
  F3_CB_1/LConn1 -- SSN Interface Block (3ph)5/RConn7
  F3_CB_1/LConn2 -- SSN Interface Block (3ph)5/RConn8
  F3_CB_1/LConn3 -- SSN Interface Block (3ph)5/RConn9
  SSN Interface Block (3ph)1/RConn2 -- F3_CB_6/LConn2
  SSN Interface Block (3ph)1/RConn1 -- F3_CB_6/LConn1
  SSN Interface Block (3ph)1/RConn3 -- F3_CB_6/LConn3
  C303/LConn1 -- F3_CB_4/RConn1
  C303/LConn2 -- F3_CB_4/RConn2
  C303/LConn3 -- F3_CB_4/RConn3
  C303/RConn2 -- 2500 kVA/LConn2
  C303/RConn3 -- 2500 kVA/LConn3
  C303/RConn1 -- 2500 kVA/LConn1
  F3_PCC/RConn1 -- F3_CB_2/LConn1 -- SSN Interface Block (3ph)5/LConn1
  F3_PCC/RConn3 -- F3_CB_2/LConn3 -- SSN Interface Block (3ph)5/LConn3
  F3_PCC/RConn2 -- F3_CB_2/LConn2 -- SSN Interface Block (3ph)5/LConn2
  500kcmil_cable/RConn2 -- opElectricFault/LConn2
  500kcmil_cable/RConn3 -- opElectricFault/LConn3
  500kcmil_cable/RConn1 -- opElectricFault/LConn1
  SSN Interface Block (3ph)2/RConn2 -- Motor/LConn2 -- F3_CB_9/LConn2
  SSN Interface Block (3ph)2/RConn3 -- Motor/LConn3 -- F3_CB_9/LConn3
  SSN Interface Block (3ph)2/RConn1 -- Motor/LConn1 -- F3_CB_9/LConn1
  PI-Section2/RConn3 -- F3_GCB/LConn3
  PI-Section2/RConn2 -- F3_GCB/LConn2
  PI-Section2/RConn1 -- F3_GCB/LConn1
  HWController_3.5MVA_NGCHP/RConn2 -- PI-Section2/LConn2
  HWController_3.5MVA_NGCHP/RConn3 -- PI-Section2/LConn3
  HWController_3.5MVA_NGCHP/RConn1 -- PI-Section2/LConn1
  1000 kVA1/RConn1 -- Critical_6/LConn1
  1000 kVA1/RConn2 -- Critical_6/LConn2
  1000 kVA1/RConn3 -- Critical_6/LConn3
  C1/RConn2 -- 6 kvar inductor at 480V  to cancel kvar produced by the stublines3/LConn2 -- B_CB_5/RConn1
  C1/RConn1 -- A_CB_5/RConn1 -- 6 kvar inductor at 480V  to cancel kvar produced by the stublines3/LConn1
  C1/RConn3 -- 6 kvar inductor at 480V  to cancel kvar produced by the stublines3/LConn3 -- C_CB_5/RConn1
  C2/RConn2 -- 6 kvar inductor at 480V  to cancel kvar produced by the stublines2/LConn2 -- B_CB_6/RConn1
  C2/RConn3 -- 6 kvar inductor at 480V  to cancel kvar produced by the stublines2/LConn3 -- C_CB_6/RConn1
  C2/RConn1 -- A_CB_6/RConn1 -- 6 kvar inductor at 480V  to cancel kvar produced by the stublines2/LConn1
  C3/RConn2 -- 6 kvar inductor at 480V  to cancel kvar produced by the stublines1/LConn2 -- B_CB_7/RConn1
  C3/RConn3 -- 6 kvar inductor at 480V  to cancel kvar produced by the stublines1/LConn3 -- C_CB_7/RConn1
  C3/RConn1 -- 6 kvar inductor at 480V  to cancel kvar produced by the stublines1/LConn1 -- A_CB_7/RConn1
  5 kvar inductor at 480V  to cancel kvar produced by the stublines/LConn1 -- C4/RConn1 -- A_CB_4/RConn1
  5 kvar inductor at 480V  to cancel kvar produced by the stublines/LConn3 -- C4/RConn3 -- C_CB_4/RConn1
  5 kvar inductor at 480V  to cancel kvar produced by the stublines/LConn2 -- C4/RConn2 -- B_CB_4/RConn1
  Three-Phase Source1/RConn3 -- PI-Section1/LConn3
  Three-Phase Source1/RConn2 -- PI-Section1/LConn2
  Three-Phase Source1/RConn1 -- PI-Section1/LConn1
  PI-Section1/RConn3 -- F3_PCC/LConn3
  PI-Section1/RConn2 -- F3_PCC/LConn2
  PI-Section1/RConn1 -- F3_PCC/LConn1
